simulink model "power_system"  (R2019a)
settings: Solver=FixedStepAuto  StartTime=0.0  StopTime=10.0  RelTol=1e-3
values from neighbouring files (symbols this model uses):
  numberOfBuses = 2    [init.m]
  numberOfGenerators = 4    [init.m]
undefined symbols (not defined in the file or in its folder): magnitude
libraries: simulink x8
(part 1 of 2)
settings Model: DataDictionary=dataHoliship.sldd  Creator=thomas.evang  LastModifiedBy=thomas.evang
settings DebuggingCC: ModelReferenceSymbolNameMessage=none
settings RTWCC: SystemTargetFile=fmu_cs2.tlc  MakeCommand=make_rtw FMIT_INTERMEDIATE_LIB_DIR=DEFAULT FMIT_ADDITIONAL_CFLAGS=  TemplateMakefile=fmu_cs2_default_tmf  Description=FMU Co-Simulation 2.0 Standalone  RetainRTWFile=on
settings STFCustomTargetCC: TargetLangStandard=C99 (ISO)  ModelReferenceCompliant=off  MATLABClassNameForMDSCustomization=Simulink.SoftwareTarget.TargetSpecificTriggerConfigurationBase  SystemTargetFile=fmu_cs2.tlc

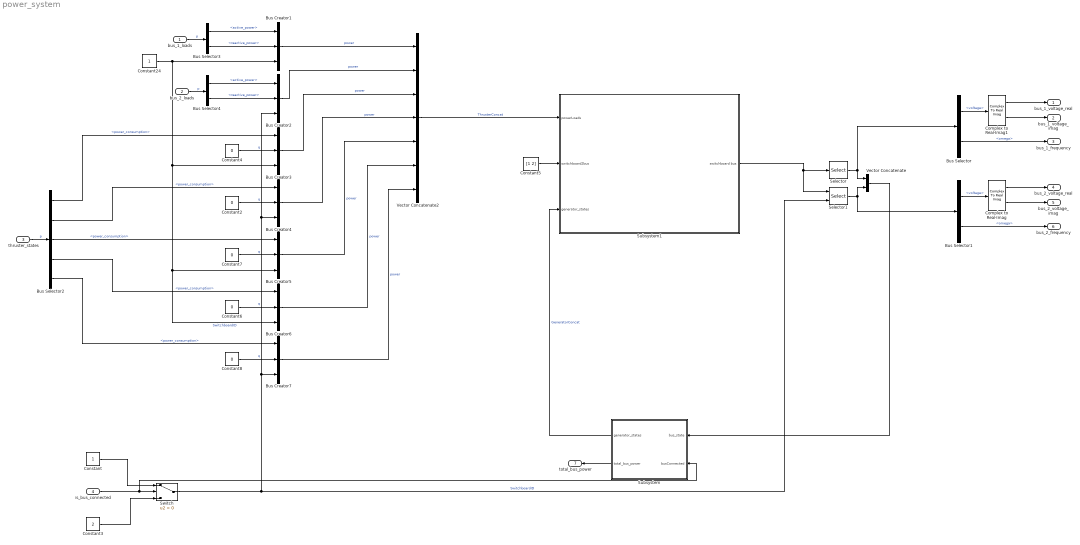
== system power_system ==
  bus_1_loads : Inport  OutDataTypeStr=Bus: bus_load
  bus_2_loads : Inport  Port=2  OutDataTypeStr=Bus: bus_load
  thruster_states : Inport  Port=3  OutDataTypeStr=Bus: thruster_states
  is_bus_connected : Inport  Port=4  OutDataTypeStr=boolean
  Bus Selector : BusSelector  OutputSignals=voltage,omega
  Bus Selector1 : BusSelector  OutputSignals=voltage,omega
  Bus Selector2 : BusSelector  OutputSignals=tunnel_thruster_1.power_consumption,tunnel_thruster_2.power_consumption,tunnel_thruster_3.power_consumption,main_propeller_port.power_consumption,main_propeller_starboard.power_consumption
  Bus Selector3 : BusSelector  OutputSignals=active_power,reactive_power
  Bus Selector4 : BusSelector  OutputSignals=active_power,reactive_power
  Bus Creator{1..7} (7 alike) : BusCreator  Inputs=3  OutDataTypeStr=Bus: powerLoadsBus  NonVirtualBus=on
      settings: InheritFromInputs=off
  Complex to Real-Imag : ComplexToRealImag
  Complex to Real-Imag1 : ComplexToRealImag
  Constant : Constant
  Constant{2,4,6..8} (5 alike) : Constant  Value=0
  Constant24 : Constant
  Constant3 : Constant  Value=2
  Constant5 : Constant  Value=[1 2]
  Selector : Selector  NumberOfDimensions=2  InputPortWidth=3  IndexOptions=Select all,Index vector (dialog)  Indices=[1 3],1  OutputSizes=1,1
  Selector1 : Selector  NumberOfDimensions=2  InputPortWidth=3  IndexOptions=Select all,Index vector (port)  Indices=[1 3],1  OutputSizes=1,1
  Subsystem : Subsystem
  Subsystem1 : Subsystem
  Switch : Switch  Criteria=u2 > Threshold
  Vector Concatenate : Concatenate  Mode=Multidimensional array  ConcatenateDimension=2
  Vector Concatenate2 : Concatenate  NumInputs=7  Mode=Multidimensional array
  bus_1_voltage_real : Outport  OutDataTypeStr=double
  bus_1_voltage_imag : Outport  Port=2  OutDataTypeStr=double
  bus_1_frequency : Outport  Port=3  OutDataTypeStr=double
  bus_2_voltage_real : Outport  Port=4  OutDataTypeStr=double
  bus_2_voltage_imag : Outport  Port=5  OutDataTypeStr=double
  bus_2_frequency : Outport  Port=6  OutDataTypeStr=double
  total_bus_power : Outport  Port=7  OutDataTypeStr=double
  wires:
  Complex to Real-Imag/1 -> bus_2_voltage_real/1
  Bus Selector2/1 -> Bus Creator3/1  "<power_consumption>"
  Bus Selector2/2 -> Bus Creator4/1  "<power_consumption>"
  Constant2/1 -> Bus Creator4/2  "q"
  Complex to Real-Imag1/2 -> bus_1_voltage_imag/1
  Bus Creator5/1 -> Vector Concatenate2/5  "power"
  Bus Creator6/1 -> Vector Concatenate2/6  "power"
  Bus Selector1/1 -> Complex to Real-Imag/1  "<voltage>"
  Bus Creator3/1 -> Vector Concatenate2/3  "power"
  Constant24/1 -> Bus Creator6/3, Bus Creator5/3, Bus Creator3/3, Bus Creator1/3  "SwitchboardID"
  Subsystem/2(total_bus_power) -> total_bus_power/1
  Vector Concatenate2/1 -> Subsystem1/1(powerLoads)  "ThrusterConcat"
  Bus Creator1/1 -> Vector Concatenate2/1  "power"
  Complex to Real-Imag/2 -> bus_2_voltage_imag/1
  Complex to Real-Imag1/1 -> bus_1_voltage_real/1
  Selector1/1 -> Vector Concatenate/2, Bus Selector1/1
  Constant5/1 -> Subsystem1/2(switchboard2bus)
  Bus Creator4/1 -> Vector Concatenate2/4  "power"
  Subsystem1/1(switchboard bus) -> Selector/1, Selector1/1
  Subsystem/1(generator_states) -> Subsystem1/3(generator_states)  "GeneratorConcat"
  Bus Selector/1 -> Complex to Real-Imag1/1  "<voltage>"
  Switch/1 -> Bus Creator2/3, Bus Creator4/3, Bus Creator7/3, Selector1/2  "SwitchboardID"
  is_bus_connected/1 -> Subsystem/2(busConnected), Switch/2
  Selector/1 -> Vector Concatenate/1, Bus Selector/1
  Vector Concatenate/1 -> Subsystem/1(bus_state)
  Constant6/1 -> Bus Creator6/2  "q"
  Bus Selector/2 -> bus_1_frequency/1  "<omega>"
  Constant8/1 -> Bus Creator7/2  "q"
  Bus Selector1/2 -> bus_2_frequency/1  "<omega>"
  Constant4/1 -> Bus Creator3/2  "q"
  Bus Creator2/1 -> Vector Concatenate2/2  "power"
  Bus Creator7/1 -> Vector Concatenate2/7  "power"
  Constant7/1 -> Bus Creator5/2  "q"
  Constant3/1 -> Switch/3
  Constant/1 -> Switch/1
  thruster_states/1 -> Bus Selector2/1  "p"
  Bus Selector2/3 -> Bus Creator5/1  "<power_consumption>"
  Bus Selector2/4 -> Bus Creator6/1  "<power_consumption>"
  Bus Selector2/5 -> Bus Creator7/1  "<power_consumption>"
  bus_1_loads/1 -> Bus Selector3/1  "p"
  Bus Selector3/1 -> Bus Creator1/1  "<active_power>"
  Bus Selector3/2 -> Bus Creator1/2  "<reactive_power>"
  bus_2_loads/1 -> Bus Selector4/1  "p"
  Bus Selector4/1 -> Bus Creator2/1  "<active_power>"
  Bus Selector4/2 -> Bus Creator2/2  "<reactive_power>"

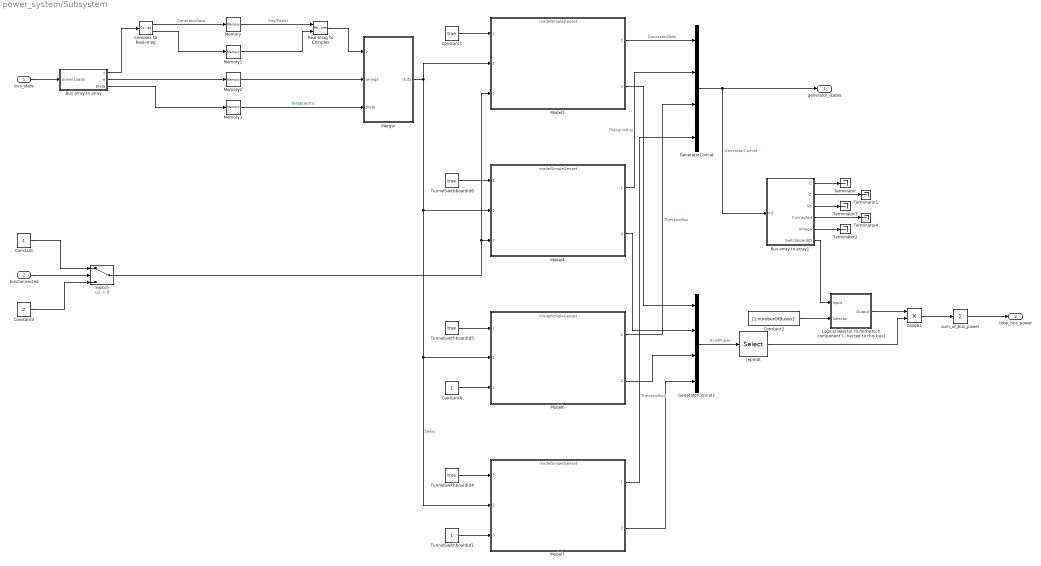
== system power_system/Subsystem ==
  bus_state : Inport
  busConnected : Inport  Port=2
  Bus array to array : Subsystem  TreatAsAtomicUnit=on
  Bus array to array1 : Subsystem  TreatAsAtomicUnit=on
  Complex to Real-Imag : ComplexToRealImag
  Constant : Constant
  Constant1 : Constant  Value=true
  Constant2 : Constant  Value=[1:numberOfBuses]'  VectorParams1D=off
  Constant3 : Constant  Value=2
  Constant6 : Constant
  Divide1 : Product
  GeneratorConcat : Concatenate  NumInputs=4  Mode=Multidimensional array
  GeneratorConcat2 : Concatenate  NumInputs=4  Mode=Multidimensional array
  Logical selector to find which component is connected to this bus1 : Subsystem
  Memory : Memory  InitialCondition=0.7
  Memory1 : Memory  InitialCondition=0.7
  Memory2 : Memory  InitialCondition=1
  Memory3 : Memory  InitialCondition=pi/4
  Merger : Subsystem  TreatAsAtomicUnit=on
  Model3 : ModelReference  ModelNameDialog=modelSimpleGenset.slx  ParameterArgumentNames=ratedPower  ParameterArgumentValues=[3000000]  UsingDefaultArgumentValue=0  SimulationMode=Normal  ModelReferenceVersion=1.210
  Model4 : ModelReference  ModelNameDialog=modelSimpleGenset.slx  ParameterArgumentNames=ratedPower  ParameterArgumentValues=3000000  UsingDefaultArgumentValue=0  SimulationMode=Normal  ModelReferenceVersion=1.210
  Model6 : ModelReference  ModelNameDialog=modelSimpleGenset.slx  ParameterArgumentNames=ratedPower  ParameterArgumentValues=3000000  UsingDefaultArgumentValue=0  SimulationMode=Normal  ModelReferenceVersion=1.210
  Model7 : ModelReference  ModelNameDialog=modelSimpleGenset.slx  ParameterArgumentNames=ratedPower  ParameterArgumentValues=3000000  UsingDefaultArgumentValue=0  SimulationMode=Normal  ModelReferenceVersion=1.210
  Real-Imag to Complex : RealImagToComplex
  Switch : Switch  Criteria=u2 > Threshold
  Terminator{,1..4} (5 alike) : Terminator
  TunnelSwithboardId1 : Constant
  TunnelSwithboardId4 : Constant  Value=true
  TunnelSwithboardId5 : Constant  Value=true
  TunnelSwithboardId6 : Constant  Value=true
  repmat : Selector  NumberOfDimensions=2  IndexOptions=Index vector (dialog),Index vector (dialog)  Indices=-1,ones(1,numberOfBuses)  OutputSizes=1,1
  sum_of_bus_power : Sum  Inputs=+  CollapseMode=Specified dimension
  generator_states : Outport
  total_bus_power : Outport  Port=2
  wires:
  Bus array to array/2(w) -> Memory2/1
  TunnelSwithboardId1/1 -> Model7/3
  Bus array to array/1(v) -> Complex to Real-Imag/1
  Real-Imag to Complex/1 -> Merger/1(v)
  Model3/1 -> GeneratorConcat/1  "GeneratorData"
  Model4/1 -> GeneratorConcat/2  "TheveninBus"
  Memory3/1 -> Merger/3(theta)  "thetaElectric"
  Merger/1(Out1) -> Model3/2, Model4/2, Model7/2, Model6/2  "Delay"
  Memory/1 -> Real-Imag to Complex/1  "RealPower"
  Memory1/1 -> Real-Imag to Complex/2
  Model6/1 -> GeneratorConcat/3  "TheveninBus"
  Memory2/1 -> Merger/2(omega)
  Model7/1 -> GeneratorConcat/4  "TheveninBus"
  Complex to Real-Imag/1 -> Memory/1  "GeneratorData"
  Complex to Real-Imag/2 -> Memory1/1
  Switch/1 -> Model4/3, Model3/3
  Bus array to array/3(theta) -> Memory3/1
  Constant6/1 -> Model6/3
  bus_state/1 -> Bus array to array/1(powerLoads)
  GeneratorConcat/1 -> Bus array to array1/1(In1), generator_states/1  "GeneratorConcat"
  Constant1/1 -> Model3/1
  TunnelSwithboardId6/1 -> Model4/1
  TunnelSwithboardId5/1 -> Model6/1
  TunnelSwithboardId4/1 -> Model7/1
  Bus array to array1/1(E) -> Terminator/1
  Bus array to array1/2(Z) -> Terminator1/1
  Bus array to array1/5(omega) -> Terminator2/1
  Bus array to array1/6(SwitchboardID) -> Logical selector to find which component is connected to this bus1/1(Input)
  Constant2/1 -> Logical selector to find which component is connected to this bus1/2(Selector)
  Model3/2 -> GeneratorConcat2/1
  Model4/2 -> GeneratorConcat2/2
  Model6/2 -> GeneratorConcat2/3
  Model7/2 -> GeneratorConcat2/4
  GeneratorConcat2/1 -> repmat/1  "AvailPower"
  Logical selector to find which component is connected to this bus1/1(Output) -> Divide1/1
  repmat/1 -> Divide1/2
  Divide1/1 -> sum_of_bus_power/1
  sum_of_bus_power/1 -> total_bus_power/1
  Bus array to array1/4(Connected) -> Terminator4/1
  Bus array to array1/3(Sb) -> Terminator3/1
  busConnected/1 -> Switch/2
  Constant/1 -> Switch/1
  Constant3/1 -> Switch/3

== system power_system/Subsystem1 ==
  powerLoads : Inport  OutDataTypeStr=Bus: powerLoadsBus  PortDimensions=[7, 1]  BusOutputAsStruct=on
  switchboard2bus : Inport  Port=2
  generator_states : Inport  Port=3  OutDataTypeStr=Bus: TheveninBus  PortDimensions=[4, 1]  BusOutputAsStruct=on
  Constant2 : Constant  Value=-1
  Integrator : Integrator
  MATLAB Function1 : MATLAB Function  Commented=on  TreatAsAtomicUnit=on
  Saturation : Saturate  UpperLimit=0  LowerLimit=-1
  Subsystem1 : Subsystem
  Subsystem2 : Subsystem
  Sum : Sum  Inputs=++|
  thrustersToBuses : Subsystem
  switchboard bus : Outport  OutDataTypeStr=Bus: swb  BusOutputAsStruct=on
  wires:
  Constant2/1 -> Sum/1
  Integrator/1 -> MATLAB Function1/1(u)
  Sum/1 -> Saturation/1
  Saturation/1 -> Integrator/1
  thrustersToBuses/1(loads) -> Subsystem2/1(loads)
  switchboard2bus/1 -> Subsystem1/1(switchboard2bus), Subsystem2/2(switchboard2bus), thrustersToBuses/2(s2b)  "s2b"
  generator_states/1 -> Subsystem1/2(Generatorset)  "Generatorset"
  Subsystem1/1(switchboard bus) -> Subsystem2/3(switchboardBus)
  Subsystem2/1(switchboard bus) -> switchboard bus/1
  Subsystem2/2(isInputValid) -> Sum/2
  powerLoads/1 -> thrustersToBuses/1(powerLoads)  "power bus"

== system power_system/Subsystem/Bus array to array ==
  powerLoads : Inport  OutDataTypeStr=Bus: swb  Partition=on  PartitionDimension=1  PartitionWidth=1  PartitionOffset=0
  Bus array to array : Subsystem  TreatAsAtomicUnit=on
  For Each : ForEach  DisableCoverage=on  IndexMode=One-based
  v : Outport  ConcatenationDimension=1
  w : Outport  Port=2  ConcatenationDimension=1
  theta : Outport  Port=3  ConcatenationDimension=1
  wires:
  powerLoads/1 -> Bus array to array/1(powerLoads)
  Bus array to array/2(w) -> w/1
  Bus array to array/3(theta) -> theta/1
  Bus array to array/1(v) -> v/1

== system power_system/Subsystem/Bus array to array1 ==
  In1 : Inport  OutDataTypeStr=Bus: TheveninBus  Partition=on  PartitionDimension=1  PartitionWidth=1  PartitionOffset=0
  Bus array to array : Subsystem  TreatAsAtomicUnit=on
  For Each : ForEach  DisableCoverage=on  IndexMode=One-based
  E : Outport  ConcatenationDimension=1
  Z : Outport  Port=2  ConcatenationDimension=1
  Sb : Outport  Port=3  ConcatenationDimension=1
  Connected : Outport  Port=4  ConcatenationDimension=1
  omega : Outport  Port=5  ConcatenationDimension=1
  SwitchboardID : Outport  Port=6  ConcatenationDimension=1
  wires:
  Bus array to array/6(SwitchboardID) -> SwitchboardID/1
  Bus array to array/5(omega) -> omega/1
  Bus array to array/4(Connected) -> Connected/1
  Bus array to array/3(Sb) -> Sb/1
  Bus array to array/1(E) -> E/1
  Bus array to array/2(Z) -> Z/1
  In1/1 -> Bus array to array/1(In1)

== system power_system/Subsystem/Logical selector to find which component is connected to this bus1 ==
  Input : Inport
  Selector : Inport  Port=2
  Relational Operator : RelationalOperator  Operator===  OutDataTypeStr=boolean  RndMeth=Simplest
  Transpose2 : Math  Operator=transpose  SaturateOnIntegerOverflow=on
  repmat : Selector  NumberOfDimensions=2  IndexOptions=Index vector (dialog),Index vector (dialog)  Indices=-1,ones(1,numberOfBuses)  OutputSizes=1,1
  repmat1 : Selector  NumberOfDimensions=2  IndexOptions=Index vector (dialog),Index vector (dialog)  Indices=-1,ones(1,numberOfGenerators)  OutputSizes=1,1
  Output : Outport
  wires:
  Transpose2/1 -> Relational Operator/2
  Relational Operator/1 -> Output/1
  repmat1/1 -> Transpose2/1
  repmat/1 -> Relational Operator/1
  Input/1 -> repmat/1
  Selector/1 -> repmat1/1

== system power_system/Subsystem/Merger ==
  v : Inport  Partition=on  PartitionDimension=1  PartitionWidth=1  PartitionOffset=0
  omega : Inport  Port=2  Partition=on  PartitionDimension=1  PartitionWidth=1  PartitionOffset=0
  theta : Inport  Port=3  Partition=on  PartitionDimension=1  PartitionWidth=1  PartitionOffset=0
  For Each : ForEach  DisableCoverage=on  IndexMode=One-based
  For Each Subsystem : Subsystem  TreatAsAtomicUnit=on
  Out1 : Outport  OutDataTypeStr=Bus: swb  ConcatenationDimension=1
  wires:
  For Each Subsystem/1(Out1) -> Out1/1
  v/1 -> For Each Subsystem/1(v)  "voltage"
  omega/1 -> For Each Subsystem/2(omega)  "omega"
  theta/1 -> For Each Subsystem/3(theta)  "thetaElectric"

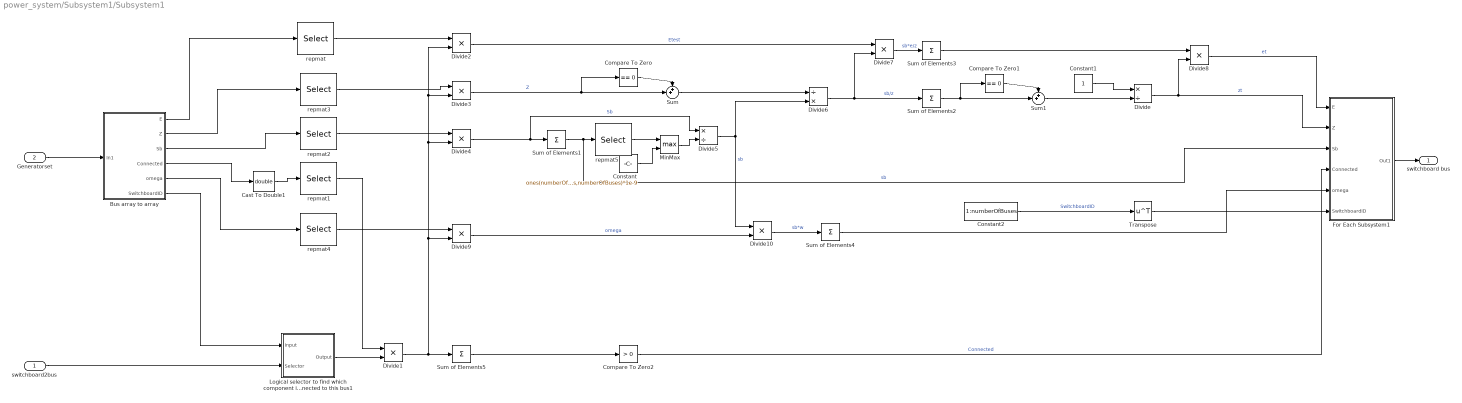
== system power_system/Subsystem1/Subsystem1 ==
  switchboard2bus : Inport
  Generatorset : Inport  Port=2  OutDataTypeStr=Bus: TheveninBus
  Bus array to array : Subsystem  TreatAsAtomicUnit=on
  Cast To Double1 : DataTypeConversion  OutDataTypeStr=double
  Compare To Zero : simulink/Logic and Bit Operations/Compare To Zero  relop===  OutDataTypeStr=uint8
  Compare To Zero1 : simulink/Logic and Bit Operations/Compare To Zero  relop===  OutDataTypeStr=uint8
  Compare To Zero2 : simulink/Logic and Bit Operations/Compare To Zero  relop=>  OutDataTypeStr=boolean
  Constant : Constant  Value=ones(numberOfGenerators,numberOfBuses)*1e-9
  Constant1 : Constant
  Constant2 : Constant  Value=1:numberOfBuses
  Divide : Product  Inputs=*/
  Divide{1..4,7..10} (8 alike) : Product
  Divide5 : Product  Inputs=*/
  Divide6 : Product  Inputs=/*
  For Each Subsystem1 : Subsystem  TreatAsAtomicUnit=on
  Logical selector to find which component is connected to this bus1 : Subsystem
  MinMax : MinMax  Function=max  Inputs=2
  Sum : Sum  Inputs=++|
  Sum of Elements{1..5} (5 alike) : Sum  Inputs=+  CollapseMode=Specified dimension
  Sum1 : Sum  Inputs=++|
  Transpose : Math  Operator=transpose  SaturateOnIntegerOverflow=on
  repmat{,1..4} (5 alike) : Selector  NumberOfDimensions=2  IndexOptions=Index vector (dialog),Index vector (dialog)  Indices=[1 2 3 4],ones(1,numberOfBuses)  OutputSizes=1,1
  repmat5 : Selector  NumberOfDimensions=2  IndexOptions=Index vector (dialog),Index vector (dialog)  Indices=ones(1,numberOfGenerators),-1  OutputSizes=1,1
  switchboard bus : Outport
  wires:
  Cast To Double1/1 -> repmat1/1
  Bus array to array/5(omega) -> repmat4/1
  Generatorset/1 -> Bus array to array/1(In1)
  For Each Subsystem1/1(Out1) -> switchboard bus/1
  Bus array to array/6(SwitchboardID) -> Logical selector to find which component is connected to this bus1/1(Input)
  Bus array to array/3(Sb) -> repmat2/1
  Bus array to array/2(Z) -> repmat3/1
  switchboard2bus/1 -> Logical selector to find which component is connected to this bus1/2(Selector)
  Logical selector to find which component is connected to this bus1/1(Output) -> Divide1/2
  Bus array to array/4(Connected) -> Cast To Double1/1
  repmat2/1 -> Divide4/1
  repmat3/1 -> Divide3/1
  repmat4/1 -> Divide9/1
  repmat1/1 -> Divide1/1
  Divide1/1 -> Divide9/2, Divide2/2, Divide3/2, Divide4/2, Sum of Elements5/1
  Divide4/1 -> Divide5/1, Sum of Elements1/1  "Sb"
  Sum of Elements1/1 -> For Each Subsystem1/3(Sb), repmat5/1  "sb"
  Divide5/1 -> Divide6/2, Divide10/1  "sb"
  repmat5/1 -> MinMax/1
  Constant/1 -> MinMax/2
  MinMax/1 -> Divide5/2
  Divide6/1 -> Divide7/2, Sum of Elements2/1  "sb/z"
  Divide3/1 -> Sum/2, Compare To Zero/1  "Z"
  Compare To Zero/1 -> Sum/1
  Sum/1 -> Divide6/1
  Sum of Elements2/1 -> Sum1/2, Compare To Zero1/1
  Compare To Zero1/1 -> Sum1/1
  Sum1/1 -> Divide/2
  Constant1/1 -> Divide/1
  Divide/1 -> Divide8/2, For Each Subsystem1/2(Z)  "zt"
  Divide7/1 -> Sum of Elements3/1  "sb*e/z"
  Divide2/1 -> Divide7/1  "Etest"
  Sum of Elements3/1 -> Divide8/1
  Divide8/1 -> For Each Subsystem1/1(E)  "et"
  Divide10/1 -> Sum of Elements4/1  "sb*w"
  Divide9/1 -> Divide10/2  "omega"
  Sum of Elements4/1 -> For Each Subsystem1/5(omega)
  Sum of Elements5/1 -> Compare To Zero2/1
  Compare To Zero2/1 -> For Each Subsystem1/4(Connected)  "Connected"
  Constant2/1 -> Transpose/1  "SwitchboardID"
  Transpose/1 -> For Each Subsystem1/6(SwitchboardID)
  Bus array to array/1(E) -> repmat/1
  repmat/1 -> Divide2/1

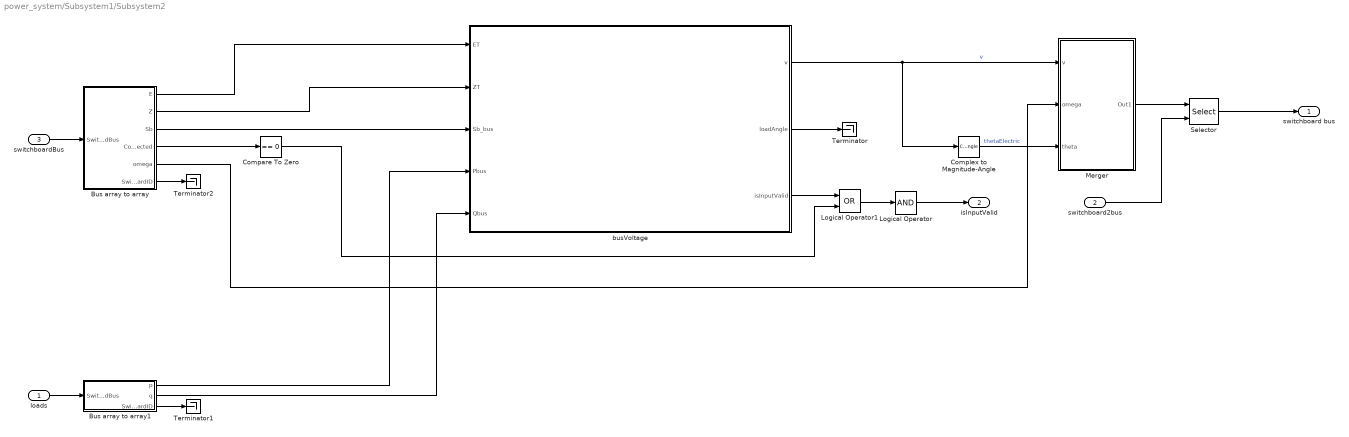
== system power_system/Subsystem1/Subsystem2 ==
  loads : Inport
  switchboard2bus : Inport  Port=2
  switchboardBus : Inport  Port=3  LockScale=on
  Bus array to array : Subsystem  TreatAsAtomicUnit=on
  Bus array to array1 : Subsystem  TreatAsAtomicUnit=on
  Compare To Zero : simulink/Logic and Bit Operations/Compare To Zero  relop===  OutDataTypeStr=boolean
  Complex to Magnitude-Angle : ComplexToMagnitudeAngle  Output=Angle
  Logical Operator : Logic  Inputs=1  AllPortsSameDT=off  OutDataTypeStr=boolean
  Logical Operator1 : Logic  Operator=OR  AllPortsSameDT=off  OutDataTypeStr=boolean
  Merger : Subsystem  TreatAsAtomicUnit=on
  Selector : Selector  InputPortWidth=numberOfBuses  IndexOptions=Index vector (port)  Indices=[1 3]  OutputSizes=1
  Terminator : Terminator
  Terminator1 : Terminator
  Terminator2 : Terminator
  busVoltage : Subsystem
  switchboard bus : Outport  OutDataTypeStr=Bus: swb
  isInputValid : Outport  Port=2
  wires:
  busVoltage/1(v) -> Merger/1(v), Complex to Magnitude-Angle/1  "v"
  busVoltage/2(loadAngle) -> Terminator/1
  Selector/1 -> switchboard bus/1
  busVoltage/3(isInputValid) -> Logical Operator1/1
  Logical Operator/1 -> isInputValid/1
  Logical Operator1/1 -> Logical Operator/1
  Complex to Magnitude-Angle/1 -> Merger/3(theta)  "thetaElectric"
  switchboard2bus/1 -> Selector/2
  Bus array to array/6(SwitchboardID) -> Terminator2/1
  Bus array to array/1(E) -> busVoltage/1(ET)
  Bus array to array/2(Z) -> busVoltage/2(ZT)
  Bus array to array/3(Sb) -> busVoltage/3(Sb_bus)
  Bus array to array/4(Connected) -> Compare To Zero/1
  loads/1 -> Bus array to array1/1(SwitchboardBus)
  switchboardBus/1 -> Bus array to array/1(SwitchboardBus)
  Bus array to array1/3(SwitchboardID) -> Terminator1/1
  Merger/1(Out1) -> Selector/1
  Compare To Zero/1 -> Logical Operator1/2
  Bus array to array/5(omega) -> Merger/2(omega)
  Bus array to array1/1(p) -> busVoltage/4(Pbus)
  Bus array to array1/2(q) -> busVoltage/5(Qbus)

== system power_system/Subsystem1/thrustersToBuses ==
  powerLoads : Inport  OutDataTypeStr=Bus: powerLoadsBus
  s2b : Inport  Port=2
  Bus array to array : Subsystem  TreatAsAtomicUnit=on
  Bus array to array1 : Subsystem  TreatAsAtomicUnit=on
  Divide : Product
  Divide1 : Product
  Logical selector to find which component is connected to this bus : Subsystem
  Sum of Elements : Sum  Inputs=+  CollapseMode=Specified dimension
  Sum of Elements1 : Sum  Inputs=+  CollapseMode=Specified dimension
  Transpose : Math  Operator=transpose  SaturateOnIntegerOverflow=on
  repmat : Selector  NumberOfDimensions=2  IndexOptions=Index vector (dialog),Index vector (dialog)  Indices=-1,ones(1,numberOfBuses)  OutputSizes=1,1
  repmat1 : Selector  NumberOfDimensions=2  IndexOptions=Index vector (dialog),Index vector (dialog)  Indices=-1,ones(1,numberOfBuses)  OutputSizes=1,1
  loads : Outport
  wires:
  Divide1/1 -> Sum of Elements1/1
  repmat1/1 -> Divide1/1
  repmat/1 -> Divide/1
  Divide/1 -> Sum of Elements/1
  Sum of Elements1/1 -> Bus array to array1/2(q)  "q"
  Bus array to array1/1(loads) -> loads/1
  powerLoads/1 -> Bus array to array/1(powerLoads)
  s2b/1 -> Transpose/1, Logical selector to find which component is connected to this bus/2(Selector)  "SwitchboardID"
  Bus array to array/3(SwitchboardID) -> Logical selector to find which component is connected to this bus/1(SwitchboardID)
  Logical selector to find which component is connected to this bus/1(Output) -> Divide/2, Divide1/2  "SwitchboardID"
  Bus array to array/1(p) -> repmat/1
  Bus array to array/2(q) -> repmat1/1
  Transpose/1 -> Bus array to array1/3(SwitchboardID)  "SwitchboardID"
  Sum of Elements/1 -> Bus array to array1/1(p)  "p"

== system power_system/Subsystem/Bus array to array/Bus array to array ==
  powerLoads : Inport  OutDataTypeStr=Bus: swb  Partition=on  PartitionDimension=2  PartitionWidth=1  PartitionOffset=0
  Bus Selector : BusSelector  OutputSignals=voltage,omega,thetaElectric
  For Each : ForEach  DisableCoverage=on  IndexMode=One-based
  v : Outport  ConcatenationDimension=2
  w : Outport  Port=2  ConcatenationDimension=2
  theta : Outport  Port=3  ConcatenationDimension=2
  wires:
  powerLoads/1 -> Bus Selector/1
  Bus Selector/2 -> w/1  "<omega>"
  Bus Selector/3 -> theta/1  "<thetaElectric>"
  Bus Selector/1 -> v/1  "<voltage>"

== system power_system/Subsystem/Bus array to array1/Bus array to array ==
  In1 : Inport  OutDataTypeStr=Bus: TheveninBus  Partition=on  PartitionDimension=2  PartitionWidth=1  PartitionOffset=0
  Bus Selector : BusSelector  OutputSignals=E,Z,Sb,Connected,omega,SwitchboardID
  For Each : ForEach  DisableCoverage=on  IndexMode=One-based
  E : Outport  ConcatenationDimension=2
  Z : Outport  Port=2  ConcatenationDimension=2
  Sb : Outport  Port=3  ConcatenationDimension=2
  Connected : Outport  Port=4  ConcatenationDimension=2
  omega : Outport  Port=5  ConcatenationDimension=2
  SwitchboardID : Outport  Port=6  ConcatenationDimension=2
  wires:
  Bus Selector/6 -> SwitchboardID/1  "<SwitchboardID>"
  Bus Selector/5 -> omega/1  "<omega>"
  Bus Selector/4 -> Connected/1  "<Connected>"
  Bus Selector/3 -> Sb/1  "<Sb>"
  Bus Selector/1 -> E/1  "<E>"
  Bus Selector/2 -> Z/1  "<Z>"
  In1/1 -> Bus Selector/1

== system power_system/Subsystem/Merger/For Each Subsystem ==
  v : Inport  Partition=on  PartitionDimension=2  PartitionWidth=1  PartitionOffset=0
  omega : Inport  Port=2  Partition=on  PartitionDimension=2  PartitionWidth=1  PartitionOffset=0
  theta : Inport  Port=3  Partition=on  PartitionDimension=2  PartitionWidth=1  PartitionOffset=0
  Bus Creator : BusCreator  Inputs=3  OutDataTypeStr=Bus: swb  NonVirtualBus=on
  For Each : ForEach  DisableCoverage=on  IndexMode=One-based
  Out1 : Outport  OutDataTypeStr=Bus: swb  ConcatenationDimension=2
  wires:
  Bus Creator/1 -> Out1/1
  v/1 -> Bus Creator/1  "voltage"
  omega/1 -> Bus Creator/2  "omega"
  theta/1 -> Bus Creator/3  "thetaElectric"

== system power_system/Subsystem1/Subsystem1/Bus array to array ==
  In1 : Inport  OutDataTypeStr=Bus: TheveninBus  Partition=on  PartitionDimension=1  PartitionWidth=1  PartitionOffset=0
  Bus array to array : Subsystem  TreatAsAtomicUnit=on
  For Each : ForEach  DisableCoverage=on  IndexMode=One-based
  E : Outport  ConcatenationDimension=1
  Z : Outport  Port=2  ConcatenationDimension=1
  Sb : Outport  Port=3  ConcatenationDimension=1
  Connected : Outport  Port=4  ConcatenationDimension=1
  omega : Outport  Port=5  ConcatenationDimension=1
  SwitchboardID : Outport  Port=6  ConcatenationDimension=1
  wires:
  Bus array to array/6(SwitchboardID) -> SwitchboardID/1
  Bus array to array/5(omega) -> omega/1
  Bus array to array/4(Connected) -> Connected/1
  Bus array to array/3(Sb) -> Sb/1
  Bus array to array/1(E) -> E/1
  Bus array to array/2(Z) -> Z/1
  In1/1 -> Bus array to array/1(In1)

== system power_system/Subsystem1/Subsystem1/For Each Subsystem1 ==
  E : Inport  Partition=on  PartitionDimension=1  PartitionWidth=1  PartitionOffset=0
  Z : Inport  Port=2  Partition=on  PartitionDimension=1  PartitionWidth=1  PartitionOffset=0
  Sb : Inport  Port=3  Partition=on  PartitionDimension=1  PartitionWidth=1  PartitionOffset=0
  Connected : Inport  Port=4  Partition=on  PartitionDimension=1  PartitionWidth=1  PartitionOffset=0
  omega : Inport  Port=5  Partition=on  PartitionDimension=1  PartitionWidth=1  PartitionOffset=0
  SwitchboardID : Inport  Port=6  Partition=on  PartitionDimension=1  PartitionWidth=1  PartitionOffset=0
  For Each : ForEach  DisableCoverage=on  IndexMode=One-based
  For Each Subsystem : Subsystem  TreatAsAtomicUnit=on
  Out1 : Outport  OutDataTypeStr=Bus: TheveninBus  ConcatenationDimension=1
  wires:
  For Each Subsystem/1(Out1) -> Out1/1
  SwitchboardID/1 -> For Each Subsystem/6(SwitchboardID)  "SwitchboardID"
  omega/1 -> For Each Subsystem/5(omega)  "omega"
  Connected/1 -> For Each Subsystem/4(Connected)  "Connected"
  Sb/1 -> For Each Subsystem/3(Sb)  "Sb"
  Z/1 -> For Each Subsystem/2(Z)  "Z"
  E/1 -> For Each Subsystem/1(E)  "E"

== system power_system/Subsystem1/Subsystem1/Logical selector to find which component is connected to this bus1 ==
  Input : Inport
  Selector : Inport  Port=2
  Relational Operator : RelationalOperator  Operator===  OutDataTypeStr=boolean  RndMeth=Simplest
  Transpose2 : Math  Operator=transpose  SaturateOnIntegerOverflow=on
  repmat : Selector  NumberOfDimensions=2  IndexOptions=Index vector (dialog),Index vector (dialog)  Indices=[1 2 3 4],ones(1,numberOfBuses)  OutputSizes=1,1
  repmat2 : Selector  NumberOfDimensions=2  IndexOptions=Index vector (dialog),Index vector (dialog)  Indices=[1 2],ones(1,numberOfGenerators)  OutputSizes=1,1
  Output : Outport
  wires:
  Transpose2/1 -> Relational Operator/2
  Relational Operator/1 -> Output/1
  Selector/1 -> repmat2/1
  repmat2/1 -> Transpose2/1
  repmat/1 -> Relational Operator/1
  Input/1 -> repmat/1

== system power_system/Subsystem1/Subsystem2/Bus array to array ==
  SwitchboardBus : Inport  OutDataTypeStr=Bus: TheveninBus  Partition=on  PartitionDimension=1  PartitionWidth=1  PartitionOffset=0
  Bus array to array2 : Subsystem  TreatAsAtomicUnit=on
  For Each : ForEach  DisableCoverage=on  IndexMode=One-based
  E : Outport  ConcatenationDimension=1
  Z : Outport  Port=2  ConcatenationDimension=1
  Sb : Outport  Port=3  ConcatenationDimension=1
  Connected : Outport  Port=4  ConcatenationDimension=1
  omega : Outport  Port=5  ConcatenationDimension=1
  SwitchboardID : Outport  Port=6  ConcatenationDimension=1
  wires:
  SwitchboardBus/1 -> Bus array to array2/1(SwitchboardBus)
  Bus array to array2/2(Z) -> Z/1
  Bus array to array2/1(E) -> E/1
  Bus array to array2/3(Sb) -> Sb/1
  Bus array to array2/4(Connected) -> Connected/1
  Bus array to array2/5(omega) -> omega/1
  Bus array to array2/6(SwitchboardID) -> SwitchboardID/1

== system power_system/Subsystem1/Subsystem2/Bus array to array1 ==
  SwitchboardBus : Inport  OutDataTypeStr=Bus: powerLoadsBus  Partition=on  PartitionDimension=1  PartitionWidth=1  PartitionOffset=0
  Bus array to array2 : Subsystem  TreatAsAtomicUnit=on
  For Each : ForEach  DisableCoverage=on  IndexMode=One-based
  p : Outport  ConcatenationDimension=1
  q : Outport  Port=2  ConcatenationDimension=1
  SwitchboardID : Outport  Port=3  ConcatenationDimension=1
  wires:
  SwitchboardBus/1 -> Bus array to array2/1(SwitchboardLoads)
  Bus array to array2/2(q) -> q/1
  Bus array to array2/1(p) -> p/1
  Bus array to array2/3(SwitchboardID) -> SwitchboardID/1

== system power_system/Subsystem1/Subsystem2/Merger ==
  v : Inport  Partition=on  PartitionDimension=1  PartitionWidth=1  PartitionOffset=0
  omega : Inport  Port=2  Partition=on  PartitionDimension=1  PartitionWidth=1  PartitionOffset=0
  theta : Inport  Port=3  Partition=on  PartitionDimension=1  PartitionWidth=1  PartitionOffset=0
  For Each : ForEach  DisableCoverage=on  IndexMode=One-based
  For Each Subsystem : Subsystem  TreatAsAtomicUnit=on
  Out1 : Outport  OutDataTypeStr=Bus: swb  ConcatenationDimension=1
  wires:
  For Each Subsystem/1(Out1) -> Out1/1
  v/1 -> For Each Subsystem/1(v)  "voltage"
  omega/1 -> For Each Subsystem/2(omega)  "omega"
  theta/1 -> For Each Subsystem/3(theta)  "thetaElectric"

== system power_system/Subsystem1/Subsystem2/busVoltage ==
  ET : Inport
  ZT : Inport  Port=2
  Sb_bus : Inport  Port=3
  Pbus : Inport  Port=4
  Qbus : Inport  Port=5
  Complex to Real-Imag : ComplexToRealImag
  Complex to Real-Imag1 : ComplexToRealImag
  Divide : Product  Inputs=*/
  Divide1 : Product  Inputs=*/
  For Iterator Subsystem1 : Subsystem  TreatAsAtomicUnit=on
  busVoltageIsValid : Subsystem
  v : Outport
  loadAngle : Outport  Port=2
  isInputValid : Outport  Port=3
  wires:
  Complex to Real-Imag1/1 -> busVoltageIsValid/6(zr)  "Zreal"
  Complex to Real-Imag1/2 -> busVoltageIsValid/5(zi)  "Zimag"
  Complex to Real-Imag/1 -> busVoltageIsValid/2(er)  "Ereal"
  Complex to Real-Imag/2 -> busVoltageIsValid/1(ei)  "Eimag"
  Sb_bus/1 -> Divide/2, Divide1/2
  Qbus/1 -> Divide1/1
  Pbus/1 -> Divide/1
  ZT/1 -> For Iterator Subsystem1/5(ZT), Complex to Real-Imag1/1  "ZT"
  Divide1/1 -> For Iterator Subsystem1/4(qbus), busVoltageIsValid/4(q)  "qbus"
  ET/1 -> For Iterator Subsystem1/1(ET), Complex to Real-Imag/1  "ET"
  Divide/1 -> For Iterator Subsystem1/3(pbus), busVoltageIsValid/3(p)  "pbus"
  For Iterator Subsystem1/1(v) -> v/1
  For Iterator Subsystem1/2(loadAngle) -> loadAngle/1
  For Iterator Subsystem1/3(isInputValid) -> isInputValid/1
  busVoltageIsValid/1(valid) -> For Iterator Subsystem1/2(valid)

== system power_system/Subsystem1/thrustersToBuses/Bus array to array ==
  powerLoads : Inport  OutDataTypeStr=Bus: powerLoadsBus  Partition=on  PartitionDimension=1  PartitionWidth=1  PartitionOffset=0
  Bus array to array : Subsystem  TreatAsAtomicUnit=on
  For Each : ForEach  DisableCoverage=on  IndexMode=One-based
  p : Outport  ConcatenationDimension=1
  q : Outport  Port=2  ConcatenationDimension=1
  SwitchboardID : Outport  Port=3  ConcatenationDimension=1
  wires:
  powerLoads/1 -> Bus array to array/1(powerLoads)
  Bus array to array/2(q) -> q/1
  Bus array to array/3(SwitchboardID) -> SwitchboardID/1
  Bus array to array/1(p) -> p/1

== system power_system/Subsystem1/thrustersToBuses/Bus array to array1 ==
  p : Inport  Partition=on  PartitionDimension=1  PartitionWidth=1  PartitionOffset=0
  q : Inport  Port=2  Partition=on  PartitionDimension=1  PartitionWidth=1  PartitionOffset=0
  SwitchboardID : Inport  Port=3  Partition=on  PartitionDimension=1  PartitionWidth=1  PartitionOffset=0
  Bus array to array1 : Subsystem  TreatAsAtomicUnit=on
  For Each : ForEach  DisableCoverage=on  IndexMode=One-based
  loads : Outport  ConcatenationDimension=1
  wires:
  p/1 -> Bus array to array1/1(p)  "p"
  q/1 -> Bus array to array1/2(q)  "q"
  SwitchboardID/1 -> Bus array to array1/3(SwitchboardID)  "SwitchboardID"
  Bus array to array1/1(loads) -> loads/1  "swb"

== system power_system/Subsystem1/thrustersToBuses/Logical selector to find which component is connected to this bus ==
  SwitchboardID : Inport
  Selector : Inport  Port=2
  Relational Operator : RelationalOperator  Operator===  OutDataTypeStr=boolean  RndMeth=Simplest
  Transpose : Math  Operator=transpose  SaturateOnIntegerOverflow=on
  repmat : Selector  NumberOfDimensions=2  IndexOptions=Index vector (dialog),Index vector (dialog)  Indices=-1,ones(1,numberOfBuses)  OutputSizes=1,1
  repmat1 : Selector  NumberOfDimensions=2  IndexOptions=Index vector (dialog),Index vector (dialog)  Indices=[1 2],ones(1,7)  OutputSizes=1,1
  Output : Outport
  wires:
  SwitchboardID/1 -> repmat/1
  repmat/1 -> Relational Operator/1
  Relational Operator/1 -> Output/1
  repmat1/1 -> Transpose/1
  Transpose/1 -> Relational Operator/2
  Selector/1 -> repmat1/1

== system power_system/Subsystem1/Subsystem1/Bus array to array/Bus array to array ==
  In1 : Inport  OutDataTypeStr=Bus: TheveninBus  Partition=on  PartitionDimension=2  PartitionWidth=1  PartitionOffset=0
  Bus Selector : BusSelector  OutputSignals=E,Z,Sb,Connected,omega,SwitchboardID
  For Each : ForEach  DisableCoverage=on  IndexMode=One-based
  E : Outport  ConcatenationDimension=2
  Z : Outport  Port=2  ConcatenationDimension=2
  Sb : Outport  Port=3  ConcatenationDimension=2
  Connected : Outport  Port=4  ConcatenationDimension=2
  omega : Outport  Port=5  ConcatenationDimension=2
  SwitchboardID : Outport  Port=6  ConcatenationDimension=2
  wires:
  Bus Selector/6 -> SwitchboardID/1  "<SwitchboardID>"
  Bus Selector/5 -> omega/1  "<omega>"
  Bus Selector/4 -> Connected/1  "<Connected>"
  Bus Selector/3 -> Sb/1  "<Sb>"
  Bus Selector/1 -> E/1  "<E>"
  Bus Selector/2 -> Z/1  "<Z>"
  In1/1 -> Bus Selector/1

== system power_system/Subsystem1/Subsystem1/For Each Subsystem1/For Each Subsystem ==
  E : Inport  Partition=on  PartitionDimension=2  PartitionWidth=1  PartitionOffset=0
  Z : Inport  Port=2  Partition=on  PartitionDimension=2  PartitionWidth=1  PartitionOffset=0
  Sb : Inport  Port=3  Partition=on  PartitionDimension=2  PartitionWidth=1  PartitionOffset=0
  Connected : Inport  Port=4  Partition=on  PartitionDimension=2  PartitionWidth=1  PartitionOffset=0
  omega : Inport  Port=5  Partition=on  PartitionDimension=2  PartitionWidth=1  PartitionOffset=0
  SwitchboardID : Inport  Port=6  Partition=on  PartitionDimension=2  PartitionWidth=1  PartitionOffset=0
  Bus Creator : BusCreator  Inputs=6  OutDataTypeStr=Bus: TheveninBus  NonVirtualBus=on
  For Each : ForEach  DisableCoverage=on  IndexMode=One-based
  Out1 : Outport  OutDataTypeStr=Bus: TheveninBus  ConcatenationDimension=2
  wires:
  Bus Creator/1 -> Out1/1
  SwitchboardID/1 -> Bus Creator/6  "SwitchboardID"
  omega/1 -> Bus Creator/5  "omega"
  Connected/1 -> Bus Creator/4  "Connected"
  Sb/1 -> Bus Creator/3  "Sb"
  Z/1 -> Bus Creator/2  "Z"
  E/1 -> Bus Creator/1  "E"

== system power_system/Subsystem1/Subsystem2/Bus array to array/Bus array to array2 ==
  SwitchboardBus : Inport  OutDataTypeStr=Bus: TheveninBus  Partition=on  PartitionDimension=2  PartitionWidth=1  PartitionOffset=0
  Bus Selector : BusSelector  OutputSignals=E,Z,Sb,Connected,omega,SwitchboardID
  For Each : ForEach  DisableCoverage=on  IndexMode=One-based
  E : Outport  ConcatenationDimension=2
  Z : Outport  Port=2  ConcatenationDimension=2
  Sb : Outport  Port=3  ConcatenationDimension=2
  Connected : Outport  Port=4  ConcatenationDimension=2
  omega : Outport  Port=5  ConcatenationDimension=2
  SwitchboardID : Outport  Port=6  ConcatenationDimension=2
  wires:
  SwitchboardBus/1 -> Bus Selector/1
  Bus Selector/2 -> Z/1  "<Z>"
  Bus Selector/1 -> E/1  "<E>"
  Bus Selector/3 -> Sb/1  "<Sb>"
  Bus Selector/4 -> Connected/1  "<Connected>"
  Bus Selector/5 -> omega/1  "<omega>"
  Bus Selector/6 -> SwitchboardID/1  "<SwitchboardID>"

== system power_system/Subsystem1/Subsystem2/Bus array to array1/Bus array to array2 ==
  SwitchboardLoads : Inport  OutDataTypeStr=Bus: powerLoadsBus  Partition=on  PartitionDimension=2  PartitionWidth=1  PartitionOffset=0
  Bus Selector : BusSelector  OutputSignals=p,q,SwitchboardID
  For Each : ForEach  DisableCoverage=on  IndexMode=One-based
  p : Outport  ConcatenationDimension=2
  q : Outport  Port=2  ConcatenationDimension=2
  SwitchboardID : Outport  Port=3  ConcatenationDimension=2
  wires:
  Bus Selector/3 -> SwitchboardID/1  "<SwitchboardID>"
  Bus Selector/2 -> q/1  "<q>"
  SwitchboardLoads/1 -> Bus Selector/1
  Bus Selector/1 -> p/1  "<p>"

== system power_system/Subsystem1/Subsystem2/Merger/For Each Subsystem ==
  v : Inport  Partition=on  PartitionDimension=2  PartitionWidth=1  PartitionOffset=0
  omega : Inport  Port=2  Partition=on  PartitionDimension=2  PartitionWidth=1  PartitionOffset=0
  theta : Inport  Port=3  Partition=on  PartitionDimension=2  PartitionWidth=1  PartitionOffset=0
  Bus Creator : BusCreator  Inputs=3  OutDataTypeStr=Bus: swb  NonVirtualBus=on
  For Each : ForEach  DisableCoverage=on  IndexMode=One-based
  Out1 : Outport  OutDataTypeStr=Bus: swb  ConcatenationDimension=2
  wires:
  Bus Creator/1 -> Out1/1
  v/1 -> Bus Creator/1  "voltage"
  omega/1 -> Bus Creator/2  "omega"
  theta/1 -> Bus Creator/3  "thetaElectric"

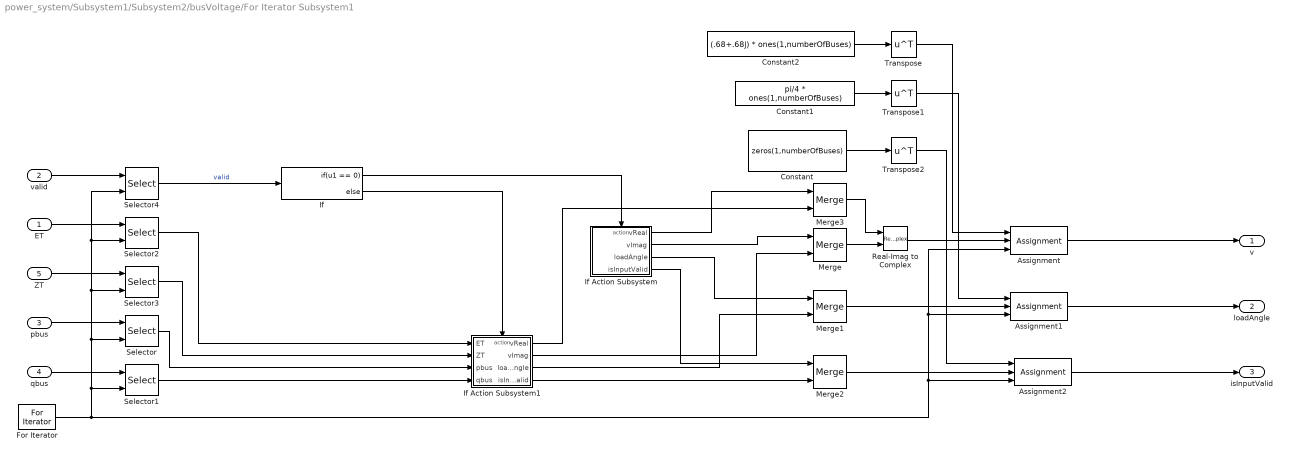
== system power_system/Subsystem1/Subsystem2/busVoltage/For Iterator Subsystem1 ==
  ET : Inport
  valid : Inport  Port=2
  pbus : Inport  Port=3
  qbus : Inport  Port=4
  ZT : Inport  Port=5
  Assignment : Assignment  NumberOfDimensions=2  DiagnosticForDimensions=Warning  IndexOptions=Assign all,Index vector (port)  Indices=1,1  OutputSizes=1,1
  Assignment1 : Assignment  NumberOfDimensions=2  DiagnosticForDimensions=Warning  IndexOptions=Assign all,Index vector (port)  Indices=1,1  OutputSizes=1,1
  Assignment2 : Assignment  NumberOfDimensions=2  DiagnosticForDimensions=Warning  IndexOptions=Assign all,Index vector (port)  Indices=1,1  OutputSizes=1,1
  Constant : Constant  Value=zeros(1,numberOfBuses)
  Constant1 : Constant  Value=pi/4 * ones(1,numberOfBuses)
  Constant2 : Constant  Value=(.68+.68j) * ones(1,numberOfBuses)
  For Iterator : ForIterator  IterationLimit=numberOfBuses
  If : If  IfExpression=u1 == 0
  If Action Subsystem : Subsystem  TreatAsAtomicUnit=on
  If Action Subsystem1 : Subsystem  TreatAsAtomicUnit=on
  Merge : Merge  InitialOutput=[0+0j]
  Merge1 : Merge
  Merge2 : Merge
  Merge3 : Merge  InitialOutput=[0+0j]
  Real-Imag to Complex : RealImagToComplex
  Selector{,1..4} (5 alike) : Selector  NumberOfDimensions=2  InputPortWidth=numberOfBuses  IndexOptions=Select all,Index vector (port)  Indices=[1 3],1  OutputSizes=1,1
  Transpose : Math  Operator=transpose  SaturateOnIntegerOverflow=on
  Transpose1 : Math  Operator=transpose  SaturateOnIntegerOverflow=on
  Transpose2 : Math  Operator=transpose  SaturateOnIntegerOverflow=on
  v : Outport
  loadAngle : Outport  Port=2
  isInputValid : Outport  Port=3
  wires:
  If Action Subsystem/4(isInputValid) -> Merge2/1
  If/2 -> If Action Subsystem1/Action
  If Action Subsystem/3(loadAngle) -> Merge1/1
  If Action Subsystem1/4(isInputValid) -> Merge2/2
  If Action Subsystem1/3(loadAngle) -> Merge1/2
  If/1 -> If Action Subsystem/Action
  ET/1 -> Selector2/1
  ZT/1 -> Selector3/1
  qbus/1 -> Selector1/1
  pbus/1 -> Selector/1
  For Iterator/1 -> Selector1/2, Selector/2, Selector3/2, Selector4/2, Selector2/2, Assignment2/3, Assignment1/3, Assignment/3
  Selector1/1 -> If Action Subsystem1/4(qbus)
  Selector/1 -> If Action Subsystem1/3(pbus)
  Selector3/1 -> If Action Subsystem1/2(ZT)
  Selector2/1 -> If Action Subsystem1/1(ET)
  Assignment/1 -> v/1
  Merge2/1 -> Assignment2/2
  Merge1/1 -> Assignment1/2
  Assignment1/1 -> loadAngle/1
  Assignment2/1 -> isInputValid/1
  valid/1 -> Selector4/1
  Real-Imag to Complex/1 -> Assignment/2
  Merge/1 -> Real-Imag to Complex/2
  Merge3/1 -> Real-Imag to Complex/1
  If Action Subsystem1/1(vReal) -> Merge3/2
  If Action Subsystem/1(vReal) -> Merge3/1
  If Action Subsystem/2(vImag) -> Merge/1
  If Action Subsystem1/2(vImag) -> Merge/2
  Constant/1 -> Transpose2/1
  Constant2/1 -> Transpose/1
  Constant1/1 -> Transpose1/1
  Transpose/1 -> Assignment/1
  Transpose1/1 -> Assignment1/1
  Transpose2/1 -> Assignment2/1
  Selector4/1 -> If/1  "valid"

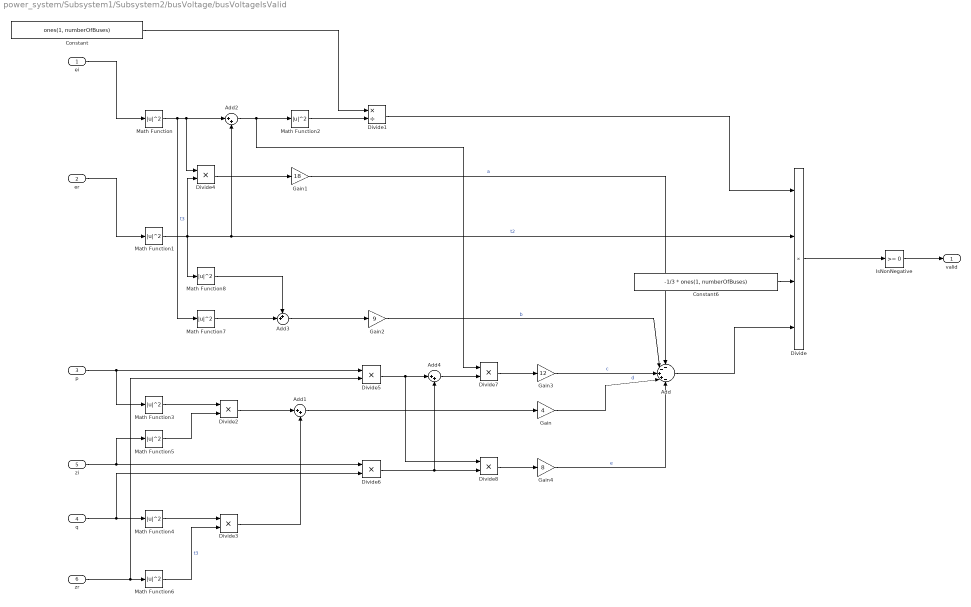
== system power_system/Subsystem1/Subsystem2/busVoltage/busVoltageIsValid ==
  ei : Inport
  er : Inport  Port=2
  p : Inport  Port=3
  q : Inport  Port=4
  zi : Inport  Port=5
  zr : Inport  Port=6
  Add : Sum  Inputs=--++-
  Add1 : Sum  Inputs=|++
  Add2 : Sum  Inputs=|++
  Add3 : Sum  Inputs=++|
  Add4 : Sum  Inputs=|++
  Constant : Constant  Value=ones(1, numberOfBuses)
  Constant6 : Constant  Value=-1/3 * ones(1, numberOfBuses)
  Divide : Product  Inputs=4
  Divide1 : Product  Inputs=*/
  Divide{2..8} (7 alike) : Product  Inputs=**
  Gain : Gain  Gain=4
  Gain1 : Gain  Gain=18
  Gain2 : Gain  Gain=9
  Gain3 : Gain  Gain=12
  Gain4 : Gain  Gain=8
  IsNonNegative : simulink/Logic and Bit Operations/Compare To Zero  relop=>=  OutDataTypeStr=boolean
  Math Function{,1..8} (9 alike) : Math  Operator=magnitude^2  SaturateOnIntegerOverflow=on
  valid : Outport
  wires:
  Math Function7/1 -> Add3/2
  Math Function8/1 -> Add3/1
  Add/1 -> Divide/4
  Gain4/1 -> Add/5  "e"
  Divide8/1 -> Gain4/1
  Gain3/1 -> Add/3  "c"
  Divide7/1 -> Gain3/1
  Add4/1 -> Divide7/2
  Gain1/1 -> Add/1  "a"
  Gain2/1 -> Add/2  "b"
  Gain/1 -> Add/4  "d"
  Divide6/1 -> Add4/2, Divide8/2
  Divide5/1 -> Add4/1, Divide8/1
  Add3/1 -> Gain2/1
  Divide4/1 -> Gain1/1
  Add1/1 -> Gain/1
  Divide3/1 -> Add1/2
  Divide2/1 -> Add1/1
  Math Function6/1 -> Divide3/2  "t3"
  Math Function4/1 -> Divide3/1
  Math Function5/1 -> Divide2/2
  Math Function3/1 -> Divide2/1
  Constant6/1 -> Divide/3
  IsNonNegative/1 -> valid/1
  zr/1 -> Math Function6/1, Divide5/2
  p/1 -> Math Function3/1, Divide5/1
  q/1 -> Divide6/2, Math Function4/1
  zi/1 -> Math Function5/1, Divide6/1
  Divide1/1 -> Divide/1
  Constant/1 -> Divide1/1
  Math Function2/1 -> Divide1/2
  Add2/1 -> Math Function2/1, Divide7/1
  Math Function/1 -> Add2/1, Divide4/1, Math Function7/1  "t3"
  Math Function1/1 -> Divide/2, Add2/2, Divide4/2, Math Function8/1  "t2"
  Divide/1 -> IsNonNegative/1
  ei/1 -> Math Function/1
  er/1 -> Math Function1/1

== system power_system/Subsystem1/thrustersToBuses/Bus array to array/Bus array to array ==
  powerLoads : Inport  OutDataTypeStr=Bus: powerLoadsBus  Partition=on  PartitionDimension=2  PartitionWidth=1  PartitionOffset=0
  Bus Selector : BusSelector  OutputSignals=p,q,SwitchboardID
  For Each : ForEach  DisableCoverage=on  IndexMode=One-based
  p : Outport  ConcatenationDimension=2
  q : Outport  Port=2  ConcatenationDimension=2
  SwitchboardID : Outport  Port=3  ConcatenationDimension=2
  wires:
  powerLoads/1 -> Bus Selector/1
  Bus Selector/2 -> q/1  "<q>"
  Bus Selector/3 -> SwitchboardID/1  "<SwitchboardID>"
  Bus Selector/1 -> p/1  "<p>"

== system power_system/Subsystem1/thrustersToBuses/Bus array to array1/Bus array to array1 ==
  p : Inport  Partition=on  PartitionDimension=2  PartitionWidth=1  PartitionOffset=0
  q : Inport  Port=2  Partition=on  PartitionDimension=2  PartitionWidth=1  PartitionOffset=0
  SwitchboardID : Inport  Port=3  Partition=on  PartitionDimension=2  PartitionWidth=1  PartitionOffset=0
  Bus Creator : BusCreator  Inputs=3  OutDataTypeStr=Bus: powerLoadsBus  NonVirtualBus=on
  For Each : ForEach  DisableCoverage=on  IndexMode=One-based
  loads : Outport  ConcatenationDimension=2
  wires:
  p/1 -> Bus Creator/1  "p"
  q/1 -> Bus Creator/2  "q"
  SwitchboardID/1 -> Bus Creator/3  "SwitchboardID"
  Bus Creator/1 -> loads/1  "swb"

== system power_system/Subsystem1/Subsystem2/busVoltage/For Iterator Subsystem1/If Action Subsystem ==
  Action Port : ActionPort  ActionPortLabel=if(u1 == 0)
  Complex to Real-Imag : ComplexToRealImag
  Constant : Constant  Value=0
  Constant1 : Constant  Value=pi/4
  Constant2 : Constant  Value=0.95
  Magnitude-Angle to Complex : MagnitudeAngleToComplex
  vReal : Outport
  vImag : Outport  Port=2
  loadAngle : Outport  Port=3
  isInputValid : Outport  Port=4
  wires:
  Constant1/1 -> loadAngle/1, Magnitude-Angle to Complex/2
  Constant2/1 -> Magnitude-Angle to Complex/1
  Constant/1 -> isInputValid/1
  Magnitude-Angle to Complex/1 -> Complex to Real-Imag/1
  Complex to Real-Imag/1 -> vReal/1
  Complex to Real-Imag/2 -> vImag/1

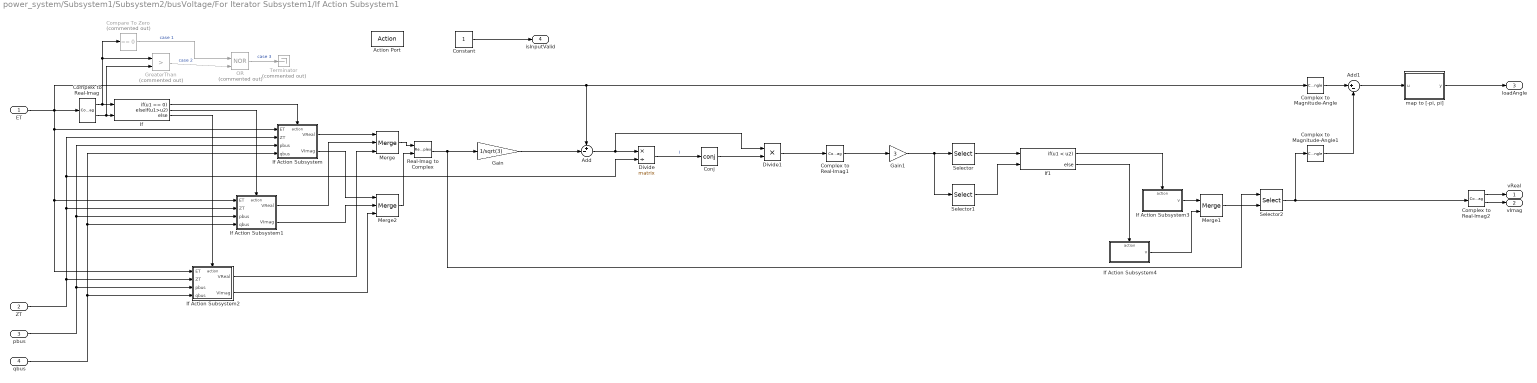
== system power_system/Subsystem1/Subsystem2/busVoltage/For Iterator Subsystem1/If Action Subsystem1 ==
  ET : Inport
  ZT : Inport  Port=2
  pbus : Inport  Port=3
  qbus : Inport  Port=4
  Action Port : ActionPort  ActionPortLabel=else
  Add : Sum  Inputs=+-|
  Add1 : Sum  Inputs=|+-
  Compare To Zero : simulink/Logic and Bit Operations/Compare To Zero  Commented=on  relop===  OutDataTypeStr=boolean
  Complex to Magnitude-Angle : ComplexToMagnitudeAngle  Output=Angle
  Complex to Magnitude-Angle1 : ComplexToMagnitudeAngle  Output=Angle
  Complex to Real-Imag : ComplexToRealImag
  Complex to Real-Imag1 : ComplexToRealImag  Output=Real
  Complex to Real-Imag2 : ComplexToRealImag
  Conj : Math  Operator=conj  SaturateOnIntegerOverflow=on
  Constant : Constant
  Divide : Product  Inputs=*/  Multiplication=Matrix(*)
  Divide1 : Product  Inputs=**
  Gain : Gain  Gain=1/sqrt(3)
  Gain1 : Gain  Gain=3
  GreaterThan : RelationalOperator  Commented=on  Operator=>  OutDataTypeStr=boolean  RndMeth=Simplest
  If : If  NumInputs=2  IfExpression=u1 == 0  ElseIfExpressions=u1>u2
  If Action Subsystem : Subsystem  TreatAsAtomicUnit=on
  If Action Subsystem1 : Subsystem  TreatAsAtomicUnit=on
  If Action Subsystem2 : Subsystem  TreatAsAtomicUnit=on
  If Action Subsystem3 : Subsystem  TreatAsAtomicUnit=on
  If Action Subsystem4 : Subsystem  TreatAsAtomicUnit=on
  If1 : If  NumInputs=2  IfExpression=u1 < u2
  Merge : Merge  Inputs=3
  Merge1 : Merge
  Merge2 : Merge  Inputs=3
  OR : Logic  Commented=on  Operator=NOR  IconShape=distinctive  AllPortsSameDT=off  OutDataTypeStr=boolean
  Real-Imag to Complex : RealImagToComplex
  Selector : Selector  InputPortWidth=2  IndexOptions=Index vector (dialog)  Indices=[1]  OutputSizes=1
  Selector1 : Selector  InputPortWidth=2  IndexOptions=Index vector (dialog)  Indices=[2]  OutputSizes=1
  Selector2 : Selector  InputPortWidth=2  IndexOptions=Index vector (port)  Indices=u1  OutputSizes=1
  Terminator : Terminator  Commented=on
  "map to [-pi, pi]" : Subsystem
  vReal : Outport
  vImag : Outport  Port=2
  loadAngle : Outport  Port=3
  isInputValid : Outport  Port=4
  wires:
  Merge1/1 -> Selector2/2
  If Action Subsystem4/1(v) -> Merge1/2
  If Action Subsystem3/1(v) -> Merge1/1
  Real-Imag to Complex/1 -> Gain/1, Selector2/1
  "map to [-pi, pi]"/1(y) -> loadAngle/1
  Add1/1 -> "map to [-pi, pi]"/1(u)
  Complex to Magnitude-Angle1/1 -> Add1/2
  Complex to Magnitude-Angle/1 -> Add1/1
  If1/2 -> If Action Subsystem4/Action
  If1/1 -> If Action Subsystem3/Action
  Selector1/1 -> If1/2
  Selector/1 -> If1/1
  Gain1/1 -> Selector/1, Selector1/1
  Complex to Real-Imag1/1 -> Gain1/1
  Divide1/1 -> Complex to Real-Imag1/1
  Add/1 -> Divide/1, Divide1/1
  Conj/1 -> Divide1/2
  Divide/1 -> Conj/1  "I"
  qbus/1 -> If Action Subsystem2/4(qbus), If Action Subsystem1/4(qbus), If Action Subsystem/4(qbus)
  pbus/1 -> If Action Subsystem2/3(pbus), If Action Subsystem1/3(pbus), If Action Subsystem/3(pbus)
  ZT/1 -> If Action Subsystem2/2(ZT), If Action Subsystem1/2(ZT), If Action Subsystem/2(ZT), Divide/2
  Gain/1 -> Add/2
  If Action Subsystem2/1(VReal) -> Merge/3
  If Action Subsystem/1(VReal) -> Merge/1
  If/3 -> If Action Subsystem2/Action
  If/2 -> If Action Subsystem1/Action
  If/1 -> If Action Subsystem/Action
  ET/1 -> Complex to Real-Imag/1, Complex to Magnitude-Angle/1, Add/1, If Action Subsystem2/1(ET), If Action Subsystem1/1(ET), If Action Subsystem/1(ET)
  Constant/1 -> isInputValid/1
  Selector2/1 -> Complex to Real-Imag2/1, Complex to Magnitude-Angle1/1
  Complex to Real-Imag2/1 -> vReal/1
  Complex to Real-Imag2/2 -> vImag/1
  If Action Subsystem/2(VImag) -> Merge2/1
  If Action Subsystem1/1(VReal) -> Merge/2
  If Action Subsystem1/2(VImag) -> Merge2/2
  If Action Subsystem2/2(VImag) -> Merge2/3
  Merge/1 -> Real-Imag to Complex/1
  Merge2/1 -> Real-Imag to Complex/2
  Complex to Real-Imag/2 -> GreaterThan/2, If/2
  Complex to Real-Imag/1 -> GreaterThan/1, Compare To Zero/1, If/1
  Compare To Zero/1 -> OR/1  "case 1"
  GreaterThan/1 -> OR/2  "case 2"
  OR/1 -> Terminator/1  "case 3"

== system power_system/Subsystem1/Subsystem2/busVoltage/For Iterator Subsystem1/If Action Subsystem1/If Action Subsystem ==
  ET : Inport
  ZT : Inport  Port=2
  pbus : Inport  Port=3
  qbus : Inport  Port=4
  Action Port : ActionPort  ActionPortLabel=if(u1 == 0)
  Add : Sum  Inputs=|++
  Complex to Real-Imag : ComplexToRealImag  Output=Imag
  Complex to Real-Imag1 : ComplexToRealImag
  Complex to Real-Imag2 : ComplexToRealImag
  Multiply : Gain  Gain=1j
  busVoltageVIzeroEr : Subsystem
  busVoltageVRzeroEr : Subsystem
  VReal : Outport
  VImag : Outport  Port=2
  wires:
  Multiply/1 -> Add/2
  busVoltageVIzeroEr/1(VI) -> Multiply/1
  Complex to Real-Imag1/1 -> busVoltageVIzeroEr/5(zr), busVoltageVRzeroEr/5(zr)
  Complex to Real-Imag1/2 -> busVoltageVIzeroEr/4(zi), busVoltageVRzeroEr/4(zi)
  qbus/1 -> busVoltageVIzeroEr/3(q), busVoltageVRzeroEr/3(q)
  pbus/1 -> busVoltageVIzeroEr/2(p), busVoltageVRzeroEr/2(p)
  Complex to Real-Imag/1 -> busVoltageVRzeroEr/1(ei), busVoltageVIzeroEr/1(ei)
  ZT/1 -> Complex to Real-Imag1/1
  ET/1 -> Complex to Real-Imag/1
  busVoltageVRzeroEr/1(VR) -> Add/1
  Add/1 -> Complex to Real-Imag2/1
  Complex to Real-Imag2/1 -> VReal/1
  Complex to Real-Imag2/2 -> VImag/1
